simulink model "V_2_0_SystemsmModelling_ModifyAirCon"  (R2020a)
settings: Solver=ode23t  StartTime=0.0  StopTime=20000  MaxStep=2000.0  RelTol=1e-3
undefined symbols (not defined in the file or in its folder): building_height, building_length, building_width, Discrete, duct_area, fan_flow_rate_table, fan_setting_table, floor_conductivity, floor_heat_transfer_coeff_internal, floor_thickness, ground_temperature, initial_temperature, roof_conductivity, roof_density, roof_heat_transfer_coeff_external, roof_heat_transfer_coeff_internal, roof_specific_heat, roof_thickness, sigbuilder_block, Time, wall_conductivity, wall_density, wall_heat_transfer_coeff_external, wall_heat_transfer_coeff_internal, wall_specific_heat, wall_thickness
libraries: fl_lib x93, nesl_utility x16, simulink x1, ctrlSharedLib x1
(part 3 of 3)

== system V_2_0_SystemsmModelling_ModifyAirCon/Room Model /Server Racks/Server Model Zone1 ==
  Heat Flow Rate Source1 : fl_lib/Thermal/Thermal Sources/Heat Flow Rate Source  heat_flow=500 W
      settings: SourceProductBaseCode=SS  InternalSimscapePortConfiguration="{\"Bottom\":[],\"Left\":[{\"id\":\"B\",\"label\":\"B\",\"type\":\"foundation.thermal.thermal\"}],\"Right\":[{\"id\":\"A\",\"label\":\"A\",\"type\":\"foundation.thermal.thermal\"}],\"Top\":[]}"
  Thermal Reference1 : fl_lib/Thermal/Thermal Elements/Thermal Reference
  Heat Flow Rate Source2 : PMIOPort  Side=Left
  connections:
  Heat Flow Rate Source1/RConn1 -- Thermal Reference1/LConn1
  Heat Flow Rate Source1/LConn1 -- Heat Flow Rate Source2/RConn1

== system V_2_0_SystemsmModelling_ModifyAirCon/Room Model /Server Racks/Server Model Zone2 ==
  Heat Flow Rate Source1 : fl_lib/Thermal/Thermal Sources/Heat Flow Rate Source  heat_flow=100 W
      settings: SourceProductBaseCode=SS  InternalSimscapePortConfiguration="{\"Bottom\":[],\"Left\":[{\"id\":\"B\",\"label\":\"B\",\"type\":\"foundation.thermal.thermal\"}],\"Right\":[{\"id\":\"A\",\"label\":\"A\",\"type\":\"foundation.thermal.thermal\"}],\"Top\":[]}"
  Thermal Reference1 : fl_lib/Thermal/Thermal Elements/Thermal Reference
  Heat Flow Rate Source2 : PMIOPort  Side=Left
  connections:
  Heat Flow Rate Source1/RConn1 -- Thermal Reference1/LConn1
  Heat Flow Rate Source1/LConn1 -- Heat Flow Rate Source2/RConn1

== system V_2_0_SystemsmModelling_ModifyAirCon/Room Model /Server Racks/Server Model Zone3 ==
  Heat Flow Rate Source1 : fl_lib/Thermal/Thermal Sources/Heat Flow Rate Source  heat_flow=500 W
      settings: SourceProductBaseCode=SS  InternalSimscapePortConfiguration="{\"Bottom\":[],\"Left\":[{\"id\":\"B\",\"label\":\"B\",\"type\":\"foundation.thermal.thermal\"}],\"Right\":[{\"id\":\"A\",\"label\":\"A\",\"type\":\"foundation.thermal.thermal\"}],\"Top\":[]}"
  Thermal Reference1 : fl_lib/Thermal/Thermal Elements/Thermal Reference
  Heat Flow Rate Source3 : PMIOPort  Side=Left
  connections:
  Heat Flow Rate Source1/RConn1 -- Thermal Reference1/LConn1
  Heat Flow Rate Source1/LConn1 -- Heat Flow Rate Source3/RConn1

== system V_2_0_SystemsmModelling_ModifyAirCon/Room Model /Server Racks/Server Model Zone4 ==
  Heat Flow Rate Source1 : fl_lib/Thermal/Thermal Sources/Heat Flow Rate Source  heat_flow=200 W
      settings: SourceProductBaseCode=SS  InternalSimscapePortConfiguration="{\"Bottom\":[],\"Left\":[{\"id\":\"B\",\"label\":\"B\",\"type\":\"foundation.thermal.thermal\"}],\"Right\":[{\"id\":\"A\",\"label\":\"A\",\"type\":\"foundation.thermal.thermal\"}],\"Top\":[]}"
  Thermal Reference1 : fl_lib/Thermal/Thermal Elements/Thermal Reference
  Heat Flow Rate Source4 : PMIOPort  Side=Left
  connections:
  Heat Flow Rate Source1/RConn1 -- Thermal Reference1/LConn1
  Heat Flow Rate Source1/LConn1 -- Heat Flow Rate Source4/RConn1

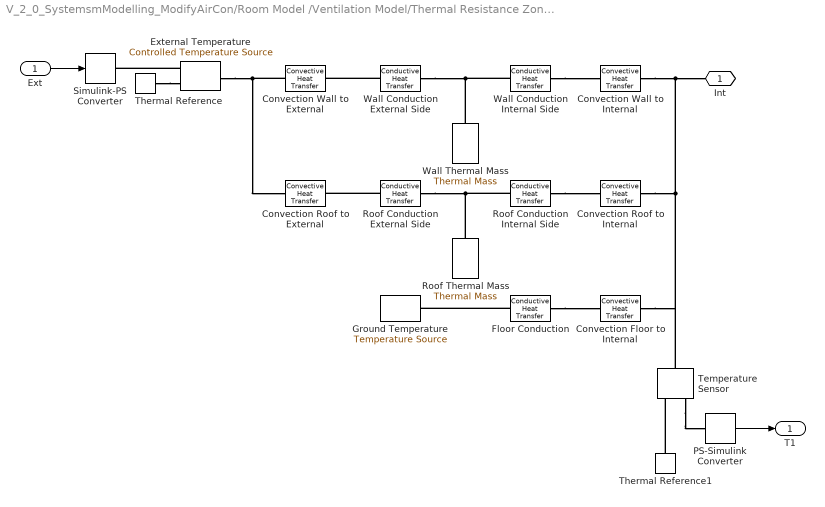
== system V_2_0_SystemsmModelling_ModifyAirCon/Room Model /Ventilation Model/Thermal Resistance Zone1 ==
  Ext : Inport
  Convection Floor to Internal : fl_lib/Thermal/Thermal Elements/Convective Heat Transfer  area=floor_area m^2  heat_tr_coeff=floor_heat_transfer_coeff_internal W/(m^2 * K)  T_specify=off  T_priority=None  T=0 K  T_nominal_specify=off  T_nominal_unit=K  T_nominal_value=1  Q_specify=off  Q_priority=None  Q=0 W  Q_nominal_specify=off  Q_nominal_unit=W  Q_nominal_value=1
  Convection Roof to External : fl_lib/Thermal/Thermal Elements/Convective Heat Transfer  area=roof_area m^2  heat_tr_coeff=roof_heat_transfer_coeff_external W/(m^2 * K)  T_specify=off  T_priority=None  T=0 K  T_nominal_specify=off  T_nominal_unit=K  T_nominal_value=1  Q_specify=off  Q_priority=None  Q=0 W  Q_nominal_specify=off  Q_nominal_unit=W  Q_nominal_value=1
  Convection Roof to Internal : fl_lib/Thermal/Thermal Elements/Convective Heat Transfer  area=roof_area m^2  heat_tr_coeff=roof_heat_transfer_coeff_internal W/(m^2 * K)  T_specify=off  T_priority=None  T=0 K  T_nominal_specify=off  T_nominal_unit=K  T_nominal_value=1  Q_specify=off  Q_priority=None  Q=0 W  Q_nominal_specify=off  Q_nominal_unit=W  Q_nominal_value=1
  Convection Wall to External : fl_lib/Thermal/Thermal Elements/Convective Heat Transfer  area=wall_area m^2  heat_tr_coeff=wall_heat_transfer_coeff_external W/(m^2 * K)  T_specify=off  T_priority=None  T=0 K  T_nominal_specify=off  T_nominal_unit=K  T_nominal_value=1  Q_specify=off  Q_priority=None  Q=0 W  Q_nominal_specify=off  Q_nominal_unit=W  Q_nominal_value=1
  Convection Wall to Internal : fl_lib/Thermal/Thermal Elements/Convective Heat Transfer  area=wall_area m^2  heat_tr_coeff=wall_heat_transfer_coeff_internal W/(m^2 * K)  T_specify=off  T_priority=None  T=0 K  T_nominal_specify=off  T_nominal_unit=K  T_nominal_value=1  Q_specify=off  Q_priority=None  Q=0 W  Q_nominal_specify=off  Q_nominal_unit=W  Q_nominal_value=1
  External Temperature : fl_lib/Thermal/Thermal Sources/Controlled Temperature Source
  Floor Conduction : fl_lib/Thermal/Thermal Elements/Conductive Heat Transfer  area=floor_area m^2  thickness=floor_thickness m  th_cond=floor_conductivity W/(m*K)  T_specify=off  T_priority=None  T=0 K  T_nominal_specify=off  T_nominal_unit=K  T_nominal_value=1  Q_specify=off  Q_priority=None  Q=0 W  Q_nominal_specify=off  Q_nominal_unit=W  Q_nominal_value=1
  Ground Temperature : fl_lib/Thermal/Thermal Sources/Temperature Source  temperature=ground_temperature degC
  PS-Simulink Converter : nesl_utility/PS-Simulink Converter  PhysicalDomain=network_engine_domain  SubClassName=ps_output  LeftPortType=input  RightPortType=output  PseudoPeriodic=off  Frequencies=[]  Unit=degC  AffineConversion=on
  Roof Conduction External Side : fl_lib/Thermal/Thermal Elements/Conductive Heat Transfer  area=roof_area m^2  thickness=roof_thickness / 2 m  th_cond=roof_conductivity W/(m*K)  T_specify=off  T_priority=None  T=0 K  T_nominal_specify=off  T_nominal_unit=K  T_nominal_value=1  Q_specify=off  Q_priority=None  Q=0 W  Q_nominal_specify=off  Q_nominal_unit=W  Q_nominal_value=1
  Roof Conduction Internal Side : fl_lib/Thermal/Thermal Elements/Conductive Heat Transfer  area=roof_area m^2  thickness=roof_thickness / 2 m  th_cond=roof_conductivity W/(m*K)  T_specify=off  T_priority=None  T=0 K  T_nominal_specify=off  T_nominal_unit=K  T_nominal_value=1  Q_specify=off  Q_priority=None  Q=0 W  Q_nominal_specify=off  Q_nominal_unit=W  Q_nominal_value=1
  Roof Thermal Mass : fl_lib/Thermal/Thermal Elements/Thermal Mass  mass=roof_area * roof_thickness * wall_density kg  sp_heat=roof_specific_heat J/kg/K  T_specify=on  T_priority=High  T=roof_initial_temperature degC  T_nominal_specify=off  T_nominal_unit=K  T_nominal_value=1  Q_specify=off  Q_priority=None  Q=0 W  Q_nominal_specify=off  Q_nominal_unit=W  Q_nominal_value=1
  Simulink-PS Converter : nesl_utility/Simulink-PS Converter  PhysicalDomain=network_engine_domain  SubClassName=ps_input  LeftPortType=input  RightPortType=output  PseudoPeriodic=off  Frequencies=[]  NoiseDistribution=none  NoiseParameters=[]  Unit=degC  AffineConversion=on  FilteringAndDerivatives=provide  SimscapeFilterOrder=1  InputFilterTimeConstant=0.001  UdotUserProvided=0
  Temperature Sensor : fl_lib/Thermal/Thermal Sensors/Temperature Sensor
  Thermal Reference : fl_lib/Thermal/Thermal Elements/Thermal Reference
  Thermal Reference1 : fl_lib/Thermal/Thermal Elements/Thermal Reference
  Wall Conduction External Side : fl_lib/Thermal/Thermal Elements/Conductive Heat Transfer  area=wall_area m^2  thickness=wall_thickness / 2 m  th_cond=wall_conductivity W/(m*K)  T_specify=off  T_priority=None  T=0 K  T_nominal_specify=off  T_nominal_unit=K  T_nominal_value=1  Q_specify=off  Q_priority=None  Q=0 W  Q_nominal_specify=off  Q_nominal_unit=W  Q_nominal_value=1
  Wall Conduction Internal Side : fl_lib/Thermal/Thermal Elements/Conductive Heat Transfer  area=wall_area m^2  thickness=wall_thickness / 2 m  th_cond=wall_conductivity W/(m*K)  T_specify=off  T_priority=None  T=0 K  T_nominal_specify=off  T_nominal_unit=K  T_nominal_value=1  Q_specify=off  Q_priority=None  Q=0 W  Q_nominal_specify=off  Q_nominal_unit=W  Q_nominal_value=1
  Wall Thermal Mass : fl_lib/Thermal/Thermal Elements/Thermal Mass  mass=wall_area * wall_thickness * wall_density kg  sp_heat=wall_specific_heat J/kg/K  T_specify=on  T_priority=High  T=wall_initial_temperature degC  T_nominal_specify=off  T_nominal_unit=K  T_nominal_value=1  Q_specify=off  Q_priority=None  Q=0 W  Q_nominal_specify=off  Q_nominal_unit=W  Q_nominal_value=1
  Int : PMIOPort  Side=Right
  T1 : Outport
  wires:
  Ext/1 -> Simulink-PS Converter/1
  PS-Simulink Converter/1 -> T1/1
  connections:
  External Temperature/RConn1 -- Simulink-PS Converter/RConn1
  Wall Conduction Internal Side/RConn1 -- Convection Wall to Internal/LConn1
  Convection Roof to Internal/RConn1 -- Convection Floor to Internal/RConn1 -- Temperature Sensor/LConn1 -- Convection Wall to Internal/RConn1 -- Int/RConn1
  External Temperature/LConn1 -- Convection Wall to External/LConn1 -- Convection Roof to External/LConn1
  Wall Conduction External Side/LConn1 -- Convection Wall to External/RConn1
  Wall Thermal Mass/LConn1 -- Wall Conduction Internal Side/LConn1 -- Wall Conduction External Side/RConn1
  Roof Thermal Mass/LConn1 -- Roof Conduction Internal Side/LConn1 -- Roof Conduction External Side/RConn1
  Roof Conduction External Side/LConn1 -- Convection Roof to External/RConn1
  Roof Conduction Internal Side/RConn1 -- Convection Roof to Internal/LConn1
  Floor Conduction/RConn1 -- Convection Floor to Internal/LConn1
  Floor Conduction/LConn1 -- Ground Temperature/LConn1
  Thermal Reference1/LConn1 -- Temperature Sensor/RConn1
  Temperature Sensor/RConn2 -- PS-Simulink Converter/LConn1
  Thermal Reference/LConn1 -- External Temperature/RConn2

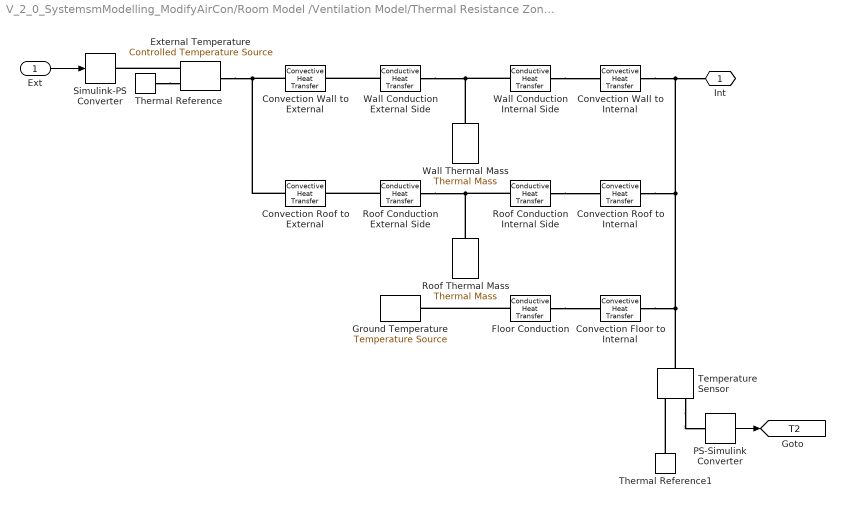
== system V_2_0_SystemsmModelling_ModifyAirCon/Room Model /Ventilation Model/Thermal Resistance Zone2 ==
  Ext : Inport
  Convection Floor to Internal : fl_lib/Thermal/Thermal Elements/Convective Heat Transfer  area=floor_area m^2  heat_tr_coeff=floor_heat_transfer_coeff_internal W/(m^2 * K)  T_specify=off  T_priority=None  T=0 K  T_nominal_specify=off  T_nominal_unit=K  T_nominal_value=1  Q_specify=off  Q_priority=None  Q=0 W  Q_nominal_specify=off  Q_nominal_unit=W  Q_nominal_value=1
  Convection Roof to External : fl_lib/Thermal/Thermal Elements/Convective Heat Transfer  area=roof_area m^2  heat_tr_coeff=roof_heat_transfer_coeff_external W/(m^2 * K)  T_specify=off  T_priority=None  T=0 K  T_nominal_specify=off  T_nominal_unit=K  T_nominal_value=1  Q_specify=off  Q_priority=None  Q=0 W  Q_nominal_specify=off  Q_nominal_unit=W  Q_nominal_value=1
  Convection Roof to Internal : fl_lib/Thermal/Thermal Elements/Convective Heat Transfer  area=roof_area m^2  heat_tr_coeff=roof_heat_transfer_coeff_internal W/(m^2 * K)  T_specify=off  T_priority=None  T=0 K  T_nominal_specify=off  T_nominal_unit=K  T_nominal_value=1  Q_specify=off  Q_priority=None  Q=0 W  Q_nominal_specify=off  Q_nominal_unit=W  Q_nominal_value=1
  Convection Wall to External : fl_lib/Thermal/Thermal Elements/Convective Heat Transfer  area=wall_area m^2  heat_tr_coeff=wall_heat_transfer_coeff_external W/(m^2 * K)  T_specify=off  T_priority=None  T=0 K  T_nominal_specify=off  T_nominal_unit=K  T_nominal_value=1  Q_specify=off  Q_priority=None  Q=0 W  Q_nominal_specify=off  Q_nominal_unit=W  Q_nominal_value=1
  Convection Wall to Internal : fl_lib/Thermal/Thermal Elements/Convective Heat Transfer  area=wall_area m^2  heat_tr_coeff=wall_heat_transfer_coeff_internal W/(m^2 * K)  T_specify=off  T_priority=None  T=0 K  T_nominal_specify=off  T_nominal_unit=K  T_nominal_value=1  Q_specify=off  Q_priority=None  Q=0 W  Q_nominal_specify=off  Q_nominal_unit=W  Q_nominal_value=1
  External Temperature : fl_lib/Thermal/Thermal Sources/Controlled Temperature Source
  Floor Conduction : fl_lib/Thermal/Thermal Elements/Conductive Heat Transfer  area=floor_area m^2  thickness=floor_thickness m  th_cond=floor_conductivity W/(m*K)  T_specify=off  T_priority=None  T=0 K  T_nominal_specify=off  T_nominal_unit=K  T_nominal_value=1  Q_specify=off  Q_priority=None  Q=0 W  Q_nominal_specify=off  Q_nominal_unit=W  Q_nominal_value=1
  Ground Temperature : fl_lib/Thermal/Thermal Sources/Temperature Source  temperature=ground_temperature degC
  PS-Simulink Converter : nesl_utility/PS-Simulink Converter  PhysicalDomain=network_engine_domain  SubClassName=ps_output  LeftPortType=input  RightPortType=output  PseudoPeriodic=off  Frequencies=[]  Unit=degC  AffineConversion=on
  Roof Conduction External Side : fl_lib/Thermal/Thermal Elements/Conductive Heat Transfer  area=roof_area m^2  thickness=roof_thickness / 2 m  th_cond=roof_conductivity W/(m*K)  T_specify=off  T_priority=None  T=0 K  T_nominal_specify=off  T_nominal_unit=K  T_nominal_value=1  Q_specify=off  Q_priority=None  Q=0 W  Q_nominal_specify=off  Q_nominal_unit=W  Q_nominal_value=1
  Roof Conduction Internal Side : fl_lib/Thermal/Thermal Elements/Conductive Heat Transfer  area=roof_area m^2  thickness=roof_thickness / 2 m  th_cond=roof_conductivity W/(m*K)  T_specify=off  T_priority=None  T=0 K  T_nominal_specify=off  T_nominal_unit=K  T_nominal_value=1  Q_specify=off  Q_priority=None  Q=0 W  Q_nominal_specify=off  Q_nominal_unit=W  Q_nominal_value=1
  Roof Thermal Mass : fl_lib/Thermal/Thermal Elements/Thermal Mass  mass=roof_area * roof_thickness * wall_density kg  sp_heat=roof_specific_heat J/kg/K  T_specify=on  T_priority=High  T=roof_initial_temperature degC  T_nominal_specify=off  T_nominal_unit=K  T_nominal_value=1  Q_specify=off  Q_priority=None  Q=0 W  Q_nominal_specify=off  Q_nominal_unit=W  Q_nominal_value=1
  Simulink-PS Converter : nesl_utility/Simulink-PS Converter  PhysicalDomain=network_engine_domain  SubClassName=ps_input  LeftPortType=input  RightPortType=output  PseudoPeriodic=off  Frequencies=[]  NoiseDistribution=none  NoiseParameters=[]  Unit=degC  AffineConversion=on  FilteringAndDerivatives=provide  SimscapeFilterOrder=1  InputFilterTimeConstant=0.001  UdotUserProvided=0
  Temperature Sensor : fl_lib/Thermal/Thermal Sensors/Temperature Sensor
  Thermal Reference : fl_lib/Thermal/Thermal Elements/Thermal Reference
  Thermal Reference1 : fl_lib/Thermal/Thermal Elements/Thermal Reference
  Wall Conduction External Side : fl_lib/Thermal/Thermal Elements/Conductive Heat Transfer  area=wall_area m^2  thickness=wall_thickness / 2 m  th_cond=wall_conductivity W/(m*K)  T_specify=off  T_priority=None  T=0 K  T_nominal_specify=off  T_nominal_unit=K  T_nominal_value=1  Q_specify=off  Q_priority=None  Q=0 W  Q_nominal_specify=off  Q_nominal_unit=W  Q_nominal_value=1
  Wall Conduction Internal Side : fl_lib/Thermal/Thermal Elements/Conductive Heat Transfer  area=wall_area m^2  thickness=wall_thickness / 2 m  th_cond=wall_conductivity W/(m*K)  T_specify=off  T_priority=None  T=0 K  T_nominal_specify=off  T_nominal_unit=K  T_nominal_value=1  Q_specify=off  Q_priority=None  Q=0 W  Q_nominal_specify=off  Q_nominal_unit=W  Q_nominal_value=1
  Wall Thermal Mass : fl_lib/Thermal/Thermal Elements/Thermal Mass  mass=wall_area * wall_thickness * wall_density kg  sp_heat=wall_specific_heat J/kg/K  T_specify=on  T_priority=High  T=wall_initial_temperature degC  T_nominal_specify=off  T_nominal_unit=K  T_nominal_value=1  Q_specify=off  Q_priority=None  Q=0 W  Q_nominal_specify=off  Q_nominal_unit=W  Q_nominal_value=1
  Int : PMIOPort  Side=Right
  tag scope: T2=global
  wires:
  PS-Simulink Converter/1 -> [T2]
  Ext/1 -> Simulink-PS Converter/1
  connections:
  Thermal Reference/LConn1 -- External Temperature/RConn2
  Temperature Sensor/RConn2 -- PS-Simulink Converter/LConn1
  Thermal Reference1/LConn1 -- Temperature Sensor/RConn1
  Floor Conduction/LConn1 -- Ground Temperature/LConn1
  Floor Conduction/RConn1 -- Convection Floor to Internal/LConn1
  Roof Conduction Internal Side/RConn1 -- Convection Roof to Internal/LConn1
  Roof Conduction External Side/LConn1 -- Convection Roof to External/RConn1
  Roof Conduction Internal Side/LConn1 -- Roof Thermal Mass/LConn1 -- Roof Conduction External Side/RConn1
  Wall Conduction Internal Side/LConn1 -- Wall Thermal Mass/LConn1 -- Wall Conduction External Side/RConn1
  Wall Conduction External Side/LConn1 -- Convection Wall to External/RConn1
  Convection Roof to External/LConn1 -- External Temperature/LConn1 -- Convection Wall to External/LConn1
  Convection Floor to Internal/RConn1 -- Int/RConn1 -- Convection Wall to Internal/RConn1 -- Convection Roof to Internal/RConn1 -- Temperature Sensor/LConn1
  Wall Conduction Internal Side/RConn1 -- Convection Wall to Internal/LConn1
  External Temperature/RConn1 -- Simulink-PS Converter/RConn1

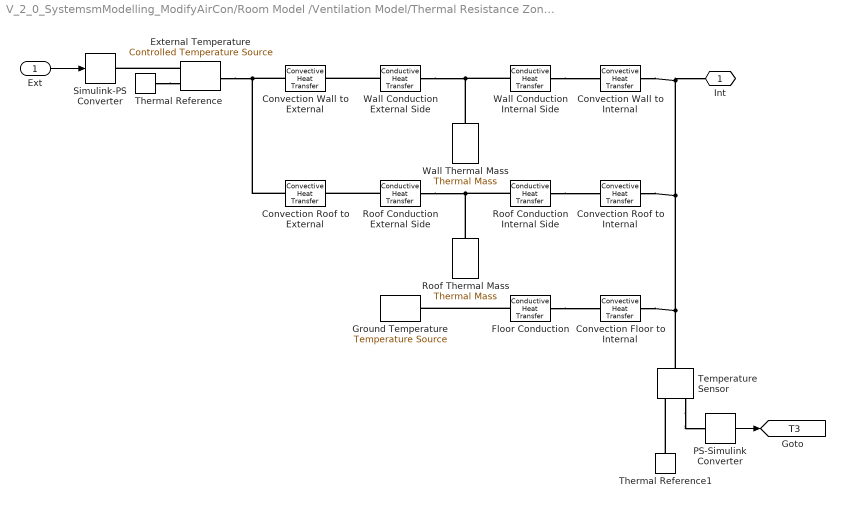
== system V_2_0_SystemsmModelling_ModifyAirCon/Room Model /Ventilation Model/Thermal Resistance Zone3 ==
  Ext : Inport
  Convection Floor to Internal : fl_lib/Thermal/Thermal Elements/Convective Heat Transfer  area=floor_area m^2  heat_tr_coeff=floor_heat_transfer_coeff_internal W/(m^2 * K)  T_specify=off  T_priority=None  T=0 K  T_nominal_specify=off  T_nominal_unit=K  T_nominal_value=1  Q_specify=off  Q_priority=None  Q=0 W  Q_nominal_specify=off  Q_nominal_unit=W  Q_nominal_value=1
  Convection Roof to External : fl_lib/Thermal/Thermal Elements/Convective Heat Transfer  area=roof_area m^2  heat_tr_coeff=roof_heat_transfer_coeff_external W/(m^2 * K)  T_specify=off  T_priority=None  T=0 K  T_nominal_specify=off  T_nominal_unit=K  T_nominal_value=1  Q_specify=off  Q_priority=None  Q=0 W  Q_nominal_specify=off  Q_nominal_unit=W  Q_nominal_value=1
  Convection Roof to Internal : fl_lib/Thermal/Thermal Elements/Convective Heat Transfer  area=roof_area m^2  heat_tr_coeff=roof_heat_transfer_coeff_internal W/(m^2 * K)  T_specify=off  T_priority=None  T=0 K  T_nominal_specify=off  T_nominal_unit=K  T_nominal_value=1  Q_specify=off  Q_priority=None  Q=0 W  Q_nominal_specify=off  Q_nominal_unit=W  Q_nominal_value=1
  Convection Wall to External : fl_lib/Thermal/Thermal Elements/Convective Heat Transfer  area=wall_area m^2  heat_tr_coeff=wall_heat_transfer_coeff_external W/(m^2 * K)  T_specify=off  T_priority=None  T=0 K  T_nominal_specify=off  T_nominal_unit=K  T_nominal_value=1  Q_specify=off  Q_priority=None  Q=0 W  Q_nominal_specify=off  Q_nominal_unit=W  Q_nominal_value=1
  Convection Wall to Internal : fl_lib/Thermal/Thermal Elements/Convective Heat Transfer  area=wall_area m^2  heat_tr_coeff=wall_heat_transfer_coeff_internal W/(m^2 * K)  T_specify=off  T_priority=None  T=0 K  T_nominal_specify=off  T_nominal_unit=K  T_nominal_value=1  Q_specify=off  Q_priority=None  Q=0 W  Q_nominal_specify=off  Q_nominal_unit=W  Q_nominal_value=1
  External Temperature : fl_lib/Thermal/Thermal Sources/Controlled Temperature Source
  Floor Conduction : fl_lib/Thermal/Thermal Elements/Conductive Heat Transfer  area=floor_area m^2  thickness=floor_thickness m  th_cond=floor_conductivity W/(m*K)  T_specify=off  T_priority=None  T=0 K  T_nominal_specify=off  T_nominal_unit=K  T_nominal_value=1  Q_specify=off  Q_priority=None  Q=0 W  Q_nominal_specify=off  Q_nominal_unit=W  Q_nominal_value=1
  Ground Temperature : fl_lib/Thermal/Thermal Sources/Temperature Source  temperature=ground_temperature degC
  PS-Simulink Converter : nesl_utility/PS-Simulink Converter  PhysicalDomain=network_engine_domain  SubClassName=ps_output  LeftPortType=input  RightPortType=output  PseudoPeriodic=off  Frequencies=[]  Unit=degC  AffineConversion=on
  Roof Conduction External Side : fl_lib/Thermal/Thermal Elements/Conductive Heat Transfer  area=roof_area m^2  thickness=roof_thickness / 2 m  th_cond=roof_conductivity W/(m*K)  T_specify=off  T_priority=None  T=0 K  T_nominal_specify=off  T_nominal_unit=K  T_nominal_value=1  Q_specify=off  Q_priority=None  Q=0 W  Q_nominal_specify=off  Q_nominal_unit=W  Q_nominal_value=1
  Roof Conduction Internal Side : fl_lib/Thermal/Thermal Elements/Conductive Heat Transfer  area=roof_area m^2  thickness=roof_thickness / 2 m  th_cond=roof_conductivity W/(m*K)  T_specify=off  T_priority=None  T=0 K  T_nominal_specify=off  T_nominal_unit=K  T_nominal_value=1  Q_specify=off  Q_priority=None  Q=0 W  Q_nominal_specify=off  Q_nominal_unit=W  Q_nominal_value=1
  Roof Thermal Mass : fl_lib/Thermal/Thermal Elements/Thermal Mass  mass=roof_area * roof_thickness * wall_density kg  sp_heat=roof_specific_heat J/kg/K  T_specify=on  T_priority=High  T=roof_initial_temperature degC  T_nominal_specify=off  T_nominal_unit=K  T_nominal_value=1  Q_specify=off  Q_priority=None  Q=0 W  Q_nominal_specify=off  Q_nominal_unit=W  Q_nominal_value=1
  Simulink-PS Converter : nesl_utility/Simulink-PS Converter  PhysicalDomain=network_engine_domain  SubClassName=ps_input  LeftPortType=input  RightPortType=output  PseudoPeriodic=off  Frequencies=[]  NoiseDistribution=none  NoiseParameters=[]  Unit=degC  AffineConversion=on  FilteringAndDerivatives=provide  SimscapeFilterOrder=1  InputFilterTimeConstant=0.001  UdotUserProvided=0
  Temperature Sensor : fl_lib/Thermal/Thermal Sensors/Temperature Sensor
  Thermal Reference : fl_lib/Thermal/Thermal Elements/Thermal Reference
  Thermal Reference1 : fl_lib/Thermal/Thermal Elements/Thermal Reference
  Wall Conduction External Side : fl_lib/Thermal/Thermal Elements/Conductive Heat Transfer  area=wall_area m^2  thickness=wall_thickness / 2 m  th_cond=wall_conductivity W/(m*K)  T_specify=off  T_priority=None  T=0 K  T_nominal_specify=off  T_nominal_unit=K  T_nominal_value=1  Q_specify=off  Q_priority=None  Q=0 W  Q_nominal_specify=off  Q_nominal_unit=W  Q_nominal_value=1
  Wall Conduction Internal Side : fl_lib/Thermal/Thermal Elements/Conductive Heat Transfer  area=wall_area m^2  thickness=wall_thickness / 2 m  th_cond=wall_conductivity W/(m*K)  T_specify=off  T_priority=None  T=0 K  T_nominal_specify=off  T_nominal_unit=K  T_nominal_value=1  Q_specify=off  Q_priority=None  Q=0 W  Q_nominal_specify=off  Q_nominal_unit=W  Q_nominal_value=1
  Wall Thermal Mass : fl_lib/Thermal/Thermal Elements/Thermal Mass  mass=wall_area * wall_thickness * wall_density kg  sp_heat=wall_specific_heat J/kg/K  T_specify=on  T_priority=High  T=wall_initial_temperature degC  T_nominal_specify=off  T_nominal_unit=K  T_nominal_value=1  Q_specify=off  Q_priority=None  Q=0 W  Q_nominal_specify=off  Q_nominal_unit=W  Q_nominal_value=1
  Int : PMIOPort  Side=Right
  tag scope: T3=global
  wires:
  Ext/1 -> Simulink-PS Converter/1
  PS-Simulink Converter/1 -> [T3]
  connections:
  External Temperature/RConn1 -- Simulink-PS Converter/RConn1
  Wall Conduction Internal Side/RConn1 -- Convection Wall to Internal/LConn1
  Temperature Sensor/LConn1 -- Convection Roof to Internal/RConn1 -- Convection Wall to Internal/RConn1 -- Int/RConn1 -- Convection Floor to Internal/RConn1
  Convection Wall to External/LConn1 -- External Temperature/LConn1 -- Convection Roof to External/LConn1
  Wall Conduction External Side/LConn1 -- Convection Wall to External/RConn1
  Wall Conduction External Side/RConn1 -- Wall Thermal Mass/LConn1 -- Wall Conduction Internal Side/LConn1
  Roof Conduction External Side/RConn1 -- Roof Thermal Mass/LConn1 -- Roof Conduction Internal Side/LConn1
  Roof Conduction External Side/LConn1 -- Convection Roof to External/RConn1
  Roof Conduction Internal Side/RConn1 -- Convection Roof to Internal/LConn1
  Floor Conduction/RConn1 -- Convection Floor to Internal/LConn1
  Floor Conduction/LConn1 -- Ground Temperature/LConn1
  Thermal Reference1/LConn1 -- Temperature Sensor/RConn1
  Temperature Sensor/RConn2 -- PS-Simulink Converter/LConn1
  Thermal Reference/LConn1 -- External Temperature/RConn2

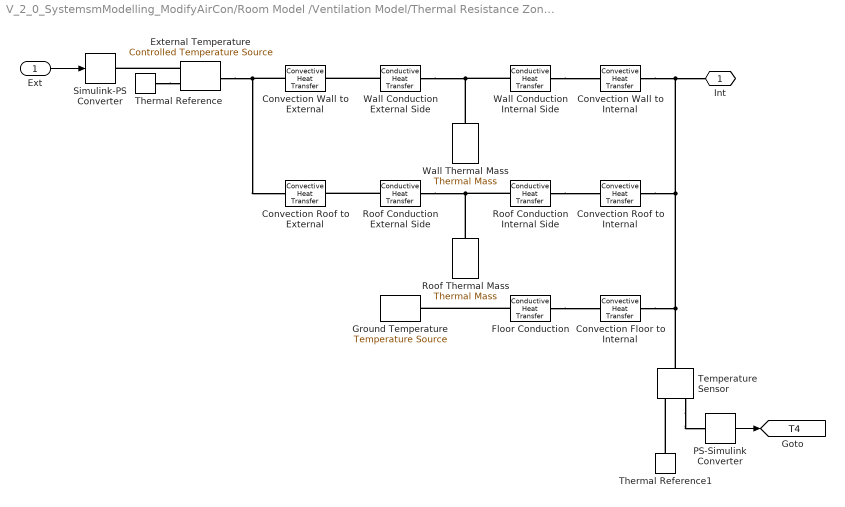
== system V_2_0_SystemsmModelling_ModifyAirCon/Room Model /Ventilation Model/Thermal Resistance Zone4 ==
  Ext : Inport
  Convection Floor to Internal : fl_lib/Thermal/Thermal Elements/Convective Heat Transfer  area=floor_area m^2  heat_tr_coeff=floor_heat_transfer_coeff_internal W/(m^2 * K)  T_specify=off  T_priority=None  T=0 K  T_nominal_specify=off  T_nominal_unit=K  T_nominal_value=1  Q_specify=off  Q_priority=None  Q=0 W  Q_nominal_specify=off  Q_nominal_unit=W  Q_nominal_value=1
  Convection Roof to External : fl_lib/Thermal/Thermal Elements/Convective Heat Transfer  area=roof_area m^2  heat_tr_coeff=roof_heat_transfer_coeff_external W/(m^2 * K)  T_specify=off  T_priority=None  T=0 K  T_nominal_specify=off  T_nominal_unit=K  T_nominal_value=1  Q_specify=off  Q_priority=None  Q=0 W  Q_nominal_specify=off  Q_nominal_unit=W  Q_nominal_value=1
  Convection Roof to Internal : fl_lib/Thermal/Thermal Elements/Convective Heat Transfer  area=roof_area m^2  heat_tr_coeff=roof_heat_transfer_coeff_internal W/(m^2 * K)  T_specify=off  T_priority=None  T=0 K  T_nominal_specify=off  T_nominal_unit=K  T_nominal_value=1  Q_specify=off  Q_priority=None  Q=0 W  Q_nominal_specify=off  Q_nominal_unit=W  Q_nominal_value=1
  Convection Wall to External : fl_lib/Thermal/Thermal Elements/Convective Heat Transfer  area=wall_area m^2  heat_tr_coeff=wall_heat_transfer_coeff_external W/(m^2 * K)  T_specify=off  T_priority=None  T=0 K  T_nominal_specify=off  T_nominal_unit=K  T_nominal_value=1  Q_specify=off  Q_priority=None  Q=0 W  Q_nominal_specify=off  Q_nominal_unit=W  Q_nominal_value=1
  Convection Wall to Internal : fl_lib/Thermal/Thermal Elements/Convective Heat Transfer  area=wall_area m^2  heat_tr_coeff=wall_heat_transfer_coeff_internal W/(m^2 * K)  T_specify=off  T_priority=None  T=0 K  T_nominal_specify=off  T_nominal_unit=K  T_nominal_value=1  Q_specify=off  Q_priority=None  Q=0 W  Q_nominal_specify=off  Q_nominal_unit=W  Q_nominal_value=1
  External Temperature : fl_lib/Thermal/Thermal Sources/Controlled Temperature Source
  Floor Conduction : fl_lib/Thermal/Thermal Elements/Conductive Heat Transfer  area=floor_area m^2  thickness=floor_thickness m  th_cond=floor_conductivity W/(m*K)  T_specify=off  T_priority=None  T=0 K  T_nominal_specify=off  T_nominal_unit=K  T_nominal_value=1  Q_specify=off  Q_priority=None  Q=0 W  Q_nominal_specify=off  Q_nominal_unit=W  Q_nominal_value=1
  Ground Temperature : fl_lib/Thermal/Thermal Sources/Temperature Source  temperature=ground_temperature degC
  PS-Simulink Converter : nesl_utility/PS-Simulink Converter  PhysicalDomain=network_engine_domain  SubClassName=ps_output  LeftPortType=input  RightPortType=output  PseudoPeriodic=off  Frequencies=[]  Unit=degC  AffineConversion=on
  Roof Conduction External Side : fl_lib/Thermal/Thermal Elements/Conductive Heat Transfer  area=roof_area m^2  thickness=roof_thickness / 2 m  th_cond=roof_conductivity W/(m*K)  T_specify=off  T_priority=None  T=0 K  T_nominal_specify=off  T_nominal_unit=K  T_nominal_value=1  Q_specify=off  Q_priority=None  Q=0 W  Q_nominal_specify=off  Q_nominal_unit=W  Q_nominal_value=1
  Roof Conduction Internal Side : fl_lib/Thermal/Thermal Elements/Conductive Heat Transfer  area=roof_area m^2  thickness=roof_thickness / 2 m  th_cond=roof_conductivity W/(m*K)  T_specify=off  T_priority=None  T=0 K  T_nominal_specify=off  T_nominal_unit=K  T_nominal_value=1  Q_specify=off  Q_priority=None  Q=0 W  Q_nominal_specify=off  Q_nominal_unit=W  Q_nominal_value=1
  Roof Thermal Mass : fl_lib/Thermal/Thermal Elements/Thermal Mass  mass=roof_area * roof_thickness * wall_density kg  sp_heat=roof_specific_heat J/kg/K  T_specify=on  T_priority=High  T=roof_initial_temperature degC  T_nominal_specify=off  T_nominal_unit=K  T_nominal_value=1  Q_specify=off  Q_priority=None  Q=0 W  Q_nominal_specify=off  Q_nominal_unit=W  Q_nominal_value=1
  Simulink-PS Converter : nesl_utility/Simulink-PS Converter  PhysicalDomain=network_engine_domain  SubClassName=ps_input  LeftPortType=input  RightPortType=output  PseudoPeriodic=off  Frequencies=[]  NoiseDistribution=none  NoiseParameters=[]  Unit=degC  AffineConversion=on  FilteringAndDerivatives=provide  SimscapeFilterOrder=1  InputFilterTimeConstant=0.001  UdotUserProvided=0
  Temperature Sensor : fl_lib/Thermal/Thermal Sensors/Temperature Sensor
  Thermal Reference : fl_lib/Thermal/Thermal Elements/Thermal Reference
  Thermal Reference1 : fl_lib/Thermal/Thermal Elements/Thermal Reference
  Wall Conduction External Side : fl_lib/Thermal/Thermal Elements/Conductive Heat Transfer  area=wall_area m^2  thickness=wall_thickness / 2 m  th_cond=wall_conductivity W/(m*K)  T_specify=off  T_priority=None  T=0 K  T_nominal_specify=off  T_nominal_unit=K  T_nominal_value=1  Q_specify=off  Q_priority=None  Q=0 W  Q_nominal_specify=off  Q_nominal_unit=W  Q_nominal_value=1
  Wall Conduction Internal Side : fl_lib/Thermal/Thermal Elements/Conductive Heat Transfer  area=wall_area m^2  thickness=wall_thickness / 2 m  th_cond=wall_conductivity W/(m*K)  T_specify=off  T_priority=None  T=0 K  T_nominal_specify=off  T_nominal_unit=K  T_nominal_value=1  Q_specify=off  Q_priority=None  Q=0 W  Q_nominal_specify=off  Q_nominal_unit=W  Q_nominal_value=1
  Wall Thermal Mass : fl_lib/Thermal/Thermal Elements/Thermal Mass  mass=wall_area * wall_thickness * wall_density kg  sp_heat=wall_specific_heat J/kg/K  T_specify=on  T_priority=High  T=wall_initial_temperature degC  T_nominal_specify=off  T_nominal_unit=K  T_nominal_value=1  Q_specify=off  Q_priority=None  Q=0 W  Q_nominal_specify=off  Q_nominal_unit=W  Q_nominal_value=1
  Int : PMIOPort  Side=Right
  tag scope: T4=global
  wires:
  PS-Simulink Converter/1 -> [T4]
  Ext/1 -> Simulink-PS Converter/1
  connections:
  Thermal Reference/LConn1 -- External Temperature/RConn2
  Temperature Sensor/RConn2 -- PS-Simulink Converter/LConn1
  Thermal Reference1/LConn1 -- Temperature Sensor/RConn1
  Floor Conduction/LConn1 -- Ground Temperature/LConn1
  Floor Conduction/RConn1 -- Convection Floor to Internal/LConn1
  Roof Conduction Internal Side/RConn1 -- Convection Roof to Internal/LConn1
  Roof Conduction External Side/LConn1 -- Convection Roof to External/RConn1
  Roof Conduction Internal Side/LConn1 -- Roof Thermal Mass/LConn1 -- Roof Conduction External Side/RConn1
  Wall Conduction Internal Side/LConn1 -- Wall Thermal Mass/LConn1 -- Wall Conduction External Side/RConn1
  Wall Conduction External Side/LConn1 -- Convection Wall to External/RConn1
  Convection Wall to External/LConn1 -- Convection Roof to External/LConn1 -- External Temperature/LConn1
  Convection Floor to Internal/RConn1 -- Int/RConn1 -- Convection Wall to Internal/RConn1 -- Convection Roof to Internal/RConn1 -- Temperature Sensor/LConn1
  Wall Conduction Internal Side/RConn1 -- Convection Wall to Internal/LConn1
  External Temperature/RConn1 -- Simulink-PS Converter/RConn1

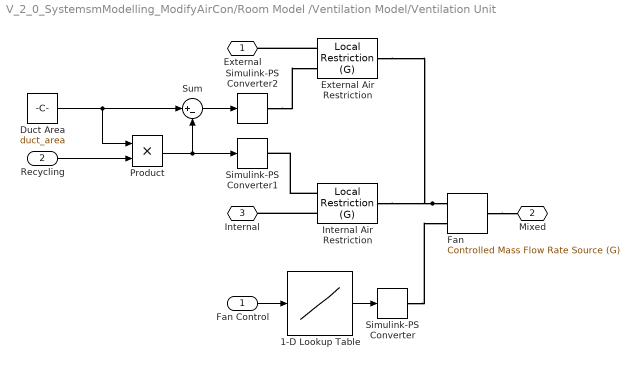
== system V_2_0_SystemsmModelling_ModifyAirCon/Room Model /Ventilation Model/Ventilation Unit ==
  Fan Control : Inport
  Recycling : Inport  Port=2
  1-D Lookup Table : Lookup_n-D  NumberOfTableDimensions=1  BreakpointsForDimension1=fan_setting_table  Table=fan_flow_rate_table  ExtrapMethod=Clip  InternalRulePriority=Speed  RndMeth=Simplest  InputSameDT=on
  Duct Area : Constant  Value=duct_area
  External Air Restriction : fl_lib/Gas/Elements/Local Restriction (G)  restriction_type=foundation.enum.restriction_type.variable  restriction_area=1e-3 m^2  min_area=1e-10 m^2  max_area=0.99 * duct_area m^2  area=duct_area m^2  Cd=0.8  B_lam=0.999
      settings: SourceProductBaseCode=SS  InternalSimscapePortConfiguration="{\"Bottom\":[],\"Left\":[{\"id\":\"A\",\"label\":\"A\",\"type\":\"foundation.gas.gas\"},{\"id\":\"area_in\",\"label\":\"AR\",\"type\":\"input\"}],\"Right\":[{\"id\":\"B\",\"label\":\"B\",\"type\":\"foundation.gas.gas\"}],\"Top\":[]}"
  Fan : fl_lib/Gas/Sources/Controlled Mass Flow Rate Source (G)  power_spec=1  area_A=duct_area m^2  area_B=duct_area m^2
      settings: SourceProductName=Foundation Library  InternalSimscapePortConfiguration="{\"Bottom\":[],\"Left\":[{\"id\":\"A\",\"label\":\"A\",\"type\":\"foundation.gas.gas\"},{\"id\":\"M\",\"label\":\"M\",\"type\":\"input\"}],\"Right\":[{\"id\":\"B\",\"label\":\"B\",\"type\":\"foundation.gas.gas\"}],\"Top\":[]}"
  Internal Air Restriction : fl_lib/Gas/Elements/Local Restriction (G)  restriction_type=foundation.enum.restriction_type.variable  restriction_area=1e-3 m^2  min_area=1e-10 m^2  max_area=0.99 * duct_area m^2  area=duct_area m^2  Cd=0.8  B_lam=0.999
      settings: SourceProductBaseCode=SS  InternalSimscapePortConfiguration="{\"Bottom\":[],\"Left\":[{\"id\":\"A\",\"label\":\"A\",\"type\":\"foundation.gas.gas\"},{\"id\":\"area_in\",\"label\":\"AR\",\"type\":\"input\"}],\"Right\":[{\"id\":\"B\",\"label\":\"B\",\"type\":\"foundation.gas.gas\"}],\"Top\":[]}"
  Product : Product
  Simulink-PS Converter : nesl_utility/Simulink-PS Converter  PhysicalDomain=network_engine_domain  SubClassName=ps_input  LeftPortType=input  RightPortType=output  PseudoPeriodic=off  Frequencies=[]  NoiseDistribution=none  NoiseParameters=[]  Unit=kg/s  AffineConversion=off  FilteringAndDerivatives=provide  SimscapeFilterOrder=1  InputFilterTimeConstant=0.001  UdotUserProvided=0
  Simulink-PS Converter1 : nesl_utility/Simulink-PS Converter  PhysicalDomain=network_engine_domain  SubClassName=ps_input  LeftPortType=input  RightPortType=output  PseudoPeriodic=off  Frequencies=[]  NoiseDistribution=none  NoiseParameters=[]  Unit=m^2  AffineConversion=off  FilteringAndDerivatives=provide  SimscapeFilterOrder=1  InputFilterTimeConstant=0.001  UdotUserProvided=0
  Simulink-PS Converter2 : nesl_utility/Simulink-PS Converter  PhysicalDomain=network_engine_domain  SubClassName=ps_input  LeftPortType=input  RightPortType=output  PseudoPeriodic=off  Frequencies=[]  NoiseDistribution=none  NoiseParameters=[]  Unit=m^2  AffineConversion=off  FilteringAndDerivatives=provide  SimscapeFilterOrder=1  InputFilterTimeConstant=0.001  UdotUserProvided=0
  Sum : Sum  Inputs=|+-
  External : PMIOPort  Side=Left
  Mixed : PMIOPort  Port=2  Side=Right
  Internal : PMIOPort  Port=3  Side=Left
  wires:
  Fan Control/1 -> 1-D Lookup Table/1
  1-D Lookup Table/1 -> Simulink-PS Converter/1
  Recycling/1 -> Product/2
  Product/1 -> Sum/2, Simulink-PS Converter1/1
  Sum/1 -> Simulink-PS Converter2/1
  Duct Area/1 -> Sum/1, Product/1
  connections:
  Fan/RConn1 -- Mixed/RConn1
  Simulink-PS Converter/RConn1 -- Fan/LConn2
  Fan/LConn1 -- Internal Air Restriction/RConn1 -- External Air Restriction/RConn1
  Internal Air Restriction/LConn2 -- Simulink-PS Converter1/RConn1
  Simulink-PS Converter2/RConn1 -- External Air Restriction/LConn2
  Internal Air Restriction/LConn1 -- Internal/RConn1
  External Air Restriction/LConn1 -- External/RConn1
